simulink model "lowpassFIR_IIR_filter"  (R2019b)
settings: Solver=VariableStepAuto  StartTime=0.0  StopTime=10.0  RelTol=1e-3
undefined symbols (not defined in the file): alpha, Fs, nb
settings Model: Creator=TarHad00  LastModifiedBy=TarHad00

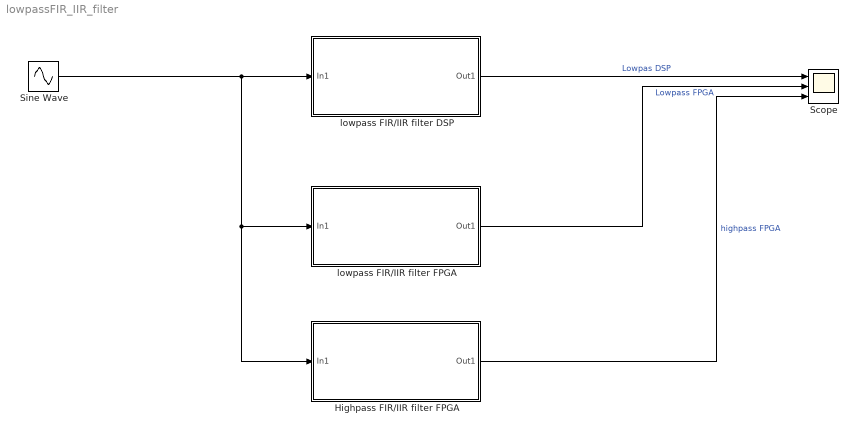
== system lowpassFIR_IIR_filter ==
  Highpass FIR/IIR filter FPGA : Subsystem
  Scope : Scope  NumInputPorts=3
  Sine Wave : Sin  Amplitude=100  Frequency=2*pi*170  SampleTime=0
  lowpass FIR/IIR filter DSP : Subsystem
  lowpass FIR/IIR filter FPGA : Subsystem
  wires:
  Sine Wave/1 -> Highpass FIR/IIR filter FPGA/1(In1), lowpass FIR/IIR filter FPGA/1(In1), lowpass FIR/IIR filter DSP/1(In1)
  lowpass FIR/IIR filter DSP/1(Out1) -> Scope/1  "Lowpas DSP"
  lowpass FIR/IIR filter FPGA/1(Out1) -> Scope/2  "Lowpass FPGA"
  Highpass FIR/IIR filter FPGA/1(Out1) -> Scope/3  "highpass FPGA"

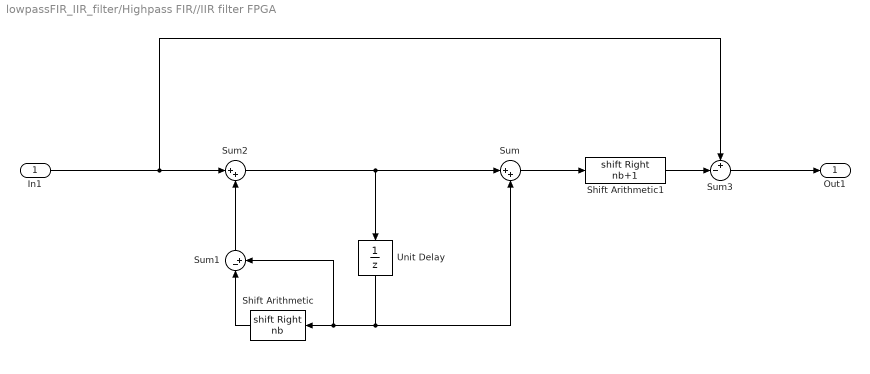
== system lowpassFIR_IIR_filter/Highpass FIR//IIR filter FPGA ==
  In1 : Inport
  Shift Arithmetic : ArithShift  BitShiftNumber=nb  BitShiftDirection=Right
  Shift Arithmetic1 : ArithShift  BitShiftNumber=nb+1  BitShiftDirection=Right
  Sum : Sum  Inputs=|++
  Sum1 : Sum  Inputs=|-+
  Sum2 : Sum  Inputs=|++
  Sum3 : Sum  Inputs=+-|
  Unit Delay : UnitDelay  SampleTime=1/Fs  HasFrameUpgradeWarning=on
  Out1 : Outport
  wires:
  Sum2/1 -> Unit Delay/1, Sum/1
  Unit Delay/1 -> Sum1/2, Shift Arithmetic/1, Sum/2
  Sum/1 -> Shift Arithmetic1/1
  In1/1 -> Sum3/1, Sum2/1
  Sum1/1 -> Sum2/2
  Shift Arithmetic/1 -> Sum1/1
  Shift Arithmetic1/1 -> Sum3/2
  Sum3/1 -> Out1/1

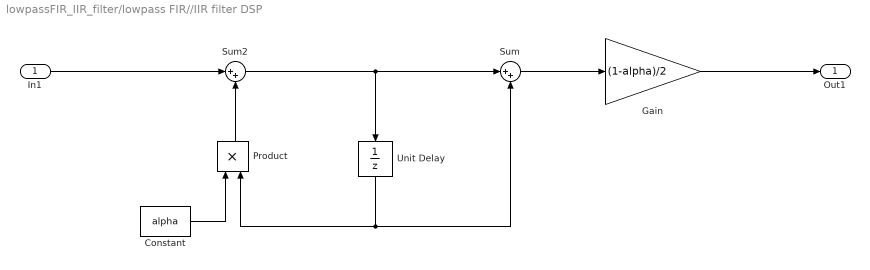
== system lowpassFIR_IIR_filter/lowpass FIR//IIR filter DSP ==
  In1 : Inport
  Constant : Constant  Value=alpha
  Gain : Gain  Gain=(1-alpha)/2
  Product : Product
  Sum : Sum  Inputs=|++
  Sum2 : Sum  Inputs=|++
  Unit Delay : UnitDelay  SampleTime=1/Fs  HasFrameUpgradeWarning=on
  Out1 : Outport
  wires:
  Sum2/1 -> Unit Delay/1, Sum/1
  Unit Delay/1 -> Product/2, Sum/2
  Product/1 -> Sum2/2
  Sum/1 -> Gain/1
  In1/1 -> Sum2/1
  Gain/1 -> Out1/1
  Constant/1 -> Product/1

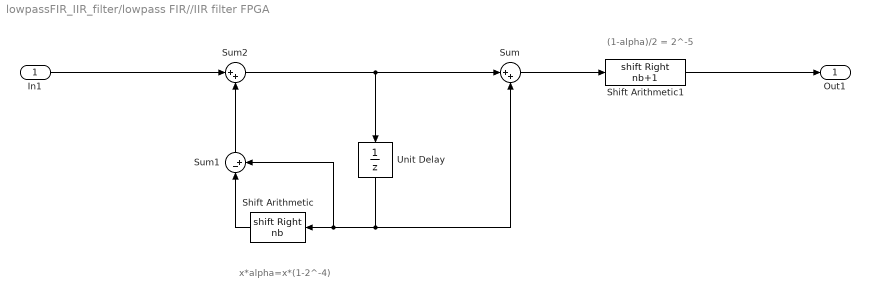
== system lowpassFIR_IIR_filter/lowpass FIR//IIR filter FPGA ==
  note: (1-alpha)/2 = 2^-5
  note: x*alpha=x*(1-2^-4)
  In1 : Inport
  Shift Arithmetic : ArithShift  BitShiftNumber=nb  BitShiftDirection=Right
  Shift Arithmetic1 : ArithShift  BitShiftNumber=nb+1  BitShiftDirection=Right
  Sum : Sum  Inputs=|++
  Sum1 : Sum  Inputs=|-+
  Sum2 : Sum  Inputs=|++
  Unit Delay : UnitDelay  SampleTime=1/Fs  HasFrameUpgradeWarning=on
  Out1 : Outport
  wires:
  Sum2/1 -> Unit Delay/1, Sum/1
  Unit Delay/1 -> Sum1/2, Shift Arithmetic/1, Sum/2
  Sum/1 -> Shift Arithmetic1/1
  In1/1 -> Sum2/1
  Shift Arithmetic1/1 -> Out1/1
  Sum1/1 -> Sum2/2
  Shift Arithmetic/1 -> Sum1/1
